simulink model "NovoModeloControlePorPressaoRevFinal_Inter"  (R2017a)
settings: Solver=ode3  StartTime=0.0  StopTime=Tsimulacao  FixedStep=Tamostra  RelTol=1e-3  EnableMultiTasking=on
values from neighbouring files (symbols this model uses):
  Delay = 0.01    [CodigoTeste.m]    (also in CodigoTesteSimulador.m = 1.5; ControlePorPressaoRevFinal.m = input('Escolha o tempo para o delay do ventilador [s] '); PlotsDaSimulacaoFinal.m = 0.05; SimulacaoFinalDaPesquisa.m = ResultadosVentiladorInterrupcaoIntermitente(i,6))
  E = 38.1970    (= 38.197)    [CodigoTeste.m]    (also in CodigoTesteSimulador.m; ControlePorPressaoRevFinal.m = 50; PlotsDaSimulacaoFinal.m = 8.33333333333; SimulacaoFinalDaPesquisa.m = 1/ResultadosVentiladorInterrupcaoIntermitente(i,5))
  Habilitar = 0    [ControlePorPressaoRevFinal.m]    (also in PlotsDaSimulacaoFinal.m = 1; SimulacaoFinalDaPesquisa.m = 1)
  Hz = 1    [ControlePorPressaoRevFinal.m]    (also in PlotsDaSimulacaoFinal.m; SimulacaoFinalDaPesquisa.m = ResultadosVentiladorInterrupcaoIntermitente(i,10))
  Limite_Vazao = 0.5    [CodigoTeste.m]    (also in ControlePorPressaoRevFinal.m = input('Escolha a vazão máxima entregue pelo o ventilador [L/; PlotsDaSimulacaoFinal.m; SimulacaoFinalDaPesquisa.m; Untitled.m = 1)
  Pasp = [-15.2979 -23.3827 -039.5964]    [CodigoTeste.m]    (also in CodigoTesteSimulador.m; ControlePorPressaoRevFinal.m = -200; PlotsDaSimulacaoFinal.m = -200; SimulacaoFinalDaPesquisa.m = -200)
  PressaoDelay = Pvent    (= 5)    [CodigoTeste.m]    (also in CodigoTesteSimulador.m; ControlePorPressaoRevFinal.m = 10; PlotsDaSimulacaoFinal.m = 10; SimulacaoFinalDaPesquisa.m = 10)
  Ptrigger = 0.0    (= 0)    [CodigoTeste.m]    (also in CodigoTesteSimulador.m = 0.5; ControlePorPressaoRevFinal.m = input('Escolha a pressão de trigger do ventilador [cmH2O] '); PlotsDaSimulacaoFinal.m = 0.5; SimulacaoFinalDaPesquisa.m = ResultadosVentiladorInterrupcaoIntermitente(i,7))
  Pvent = 5    [CodigoTeste.m]    (also in CodigoTesteSimulador.m; ControlePorPressaoRevFinal.m = 10; PlotsDaSimulacaoFinal.m = 10; SimulacaoFinalDaPesquisa.m = 10)
  Rrs = 3.3464    [CodigoTeste.m]    (also in CodigoTesteSimulador.m; ControlePorPressaoRevFinal.m = 5; PlotsDaSimulacaoFinal.m = 5; SimulacaoFinalDaPesquisa.m = ResultadosVentiladorInterrupcaoIntermitente(i,4))
  Tamanho_Sonda = 10    [CodigoTeste.m]    (also in CodigoTesteSimulador.m; ControlePorPressaoRevFinal.m = input('Qual o tamanho da sonda utilizada [FR]? 00, 06, 08, 1; PlotsDaSimulacaoFinal.m = 6; SimulacaoFinalDaPesquisa.m = ResultadosVentiladorInterrupcaoIntermitente(i,9))
  TOT = 7.5    [CodigoTeste.m]    (also in CodigoTesteSimulador.m; ControlePorPressaoRevFinal.m = input('Qual o tamanho do Tubo Orotraquial utilizado [mm]? 7.; PlotsDaSimulacaoFinal.m; SimulacaoFinalDaPesquisa.m = ResultadosVentiladorInterrupcaoIntermitente(i,8))
  VolumeInicial = VR+PressaoInicial/E    (= 0.130900332487)    [CodigoTeste.m]    (also in CodigoTesteSimulador.m; ControlePorPressaoRevFinal.m = 1.4; PlotsDaSimulacaoFinal.m = 2.4; SimulacaoFinalDaPesquisa.m = 2.4)
  VR = 0    [CodigoTeste.m]    (also in CodigoTesteSimulador.m; ControlePorPressaoRevFinal.m = 1.2; PlotsDaSimulacaoFinal.m = 1.2; SimulacaoFinalDaPesquisa.m = 1.2)
libraries: simulink x2
settings Model: Creator=Proprietário  LastModifiedBy=Texugão
settings DataIOCC: LimitDataPoints=on  SaveFormat=Array
settings OptimizationCC: LifeSpan=inf
settings DebuggingCC: SolverPrmCheckMsg=warning  SFUnexpectedBacktrackingDiag=warning  SFNoUnconditionalDefaultTransitionDiag=warning  SFExecutionAtInitializationDiag=none
settings HardwareCC: ProdBitPerPointer=32  ProdBitPerSizeT=32  ProdBitPerPtrDiffT=32  ProdLargestAtomicFloat=None  ProdIntDivRoundTo=Undefined  ProdEndianess=Unspecified  ProdWordSize=32  ProdHWDeviceType=32-bit Generic
settings ModelReferenceCC: PropagateSignalLabelsOutOfModel=off
settings GRTTargetCC: TargetLangStandard=C89/C90 (ANSI)  GeneratePreprocessorConditionals=Disable all
settings ConfigComp: CovMetricSettings=dw  CovHtmlReporting=on  CovSaveCumulativeToWorkspaceVar=on  CovSaveSingleToWorkspaceVar=on  CovExternalEMLEnable=off  CovSFcnEnable=off

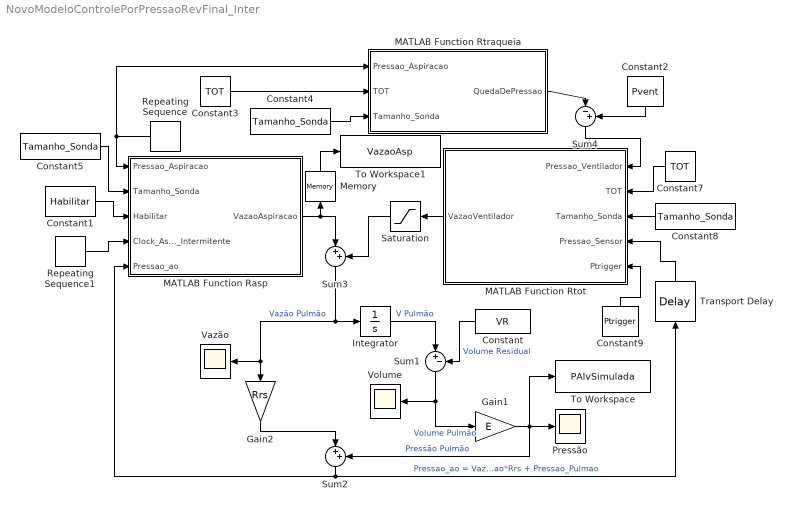
== system NovoModeloControlePorPressaoRevFinal_Inter ==
  Constant : Constant  Value=VR
  Constant1 : Constant  Value=Habilitar
  Constant2 : Constant  Value=Pvent
  Constant3 : Constant  Value=TOT
  Constant4 : Constant  Value=Tamanho_Sonda
  Constant5 : Constant  Value=Tamanho_Sonda
  Constant7 : Constant  Value=TOT
  Constant8 : Constant  Value=Tamanho_Sonda
  Constant9 : Constant  Value=Ptrigger
  Gain1 : Gain  Gain=E
  Gain2 : Gain  Gain=Rrs
  Integrator : Integrator  InitialCondition=VolumeInicial
  MATLAB Function Rasp : MATLAB Function  TreatAsAtomicUnit=on
  MATLAB Function Rtot : MATLAB Function  TreatAsAtomicUnit=on
  MATLAB Function Rtraqueia : MATLAB Function  TreatAsAtomicUnit=on
  Memory : Memory
  Pressão : Scope
  Repeating Sequence : simulink/Sources/Repeating Sequence  rep_seq_t=[0 60 60.001 75 75.001 95]  rep_seq_y=[0 0 Pasp Pasp 0 0]
  Repeating Sequence1 : simulink/Sources/Repeating Sequence  rep_seq_t=[0 1/Hz 1/Hz+0.001 2/Hz]  rep_seq_y=[1 1 0 0]
  Saturation : Saturate  UpperLimit=Limite_Vazao  LowerLimit=-Limite_Vazao
  Sum1 : Sum  Inputs=|+-
  Sum2 : Sum  Inputs=|++
  Sum3 : Sum  Inputs=|++
  Sum4 : Sum  Inputs=|-+
  To Workspace : ToWorkspace  VariableName=PAlvSimulada  SaveFormat=Timeseries  SampleTime=-1
  To Workspace1 : ToWorkspace  VariableName=VazaoAsp  SaveFormat=Timeseries  SampleTime=-1
  Transport Delay : TransportDelay  DelayTime=Delay  InitialOutput=PressaoDelay
  Vazão : Scope
  Volume : Scope
  wires:
  Integrator/1 -> Sum1/1  "V Pulmão"
  Constant/1 -> Sum1/2  "Volume Residual"
  Sum3/1 -> Integrator/1, Vazão/1, Gain2/1  "Vazão Pulmão"
  Sum1/1 -> Gain1/1, Volume/1  "Volume Pulmão"
  Constant5/1 -> MATLAB Function Rasp/2(Tamanho_Sonda)
  Constant8/1 -> MATLAB Function Rtot/3(Tamanho_Sonda)
  Constant7/1 -> MATLAB Function Rtot/2(TOT)
  Transport Delay/1 -> MATLAB Function Rtot/4(Pressao_Sensor)
  Constant9/1 -> MATLAB Function Rtot/5(Ptrigger)
  MATLAB Function Rasp/1(VazaoAspiracao) -> Sum3/1, Memory/1
  Gain1/1 -> To Workspace/1, Pressão/1, Sum2/2  "Pressão Pulmão"
  Gain2/1 -> Sum2/1
  Sum2/1 -> MATLAB Function Rasp/5(Pressao_ao), Transport Delay/1  "Pressao_ao = Vazao_Pulmao*Rrs + Pressao_Pulmao"
  MATLAB Function Rtot/1(VazaoVentilador) -> Saturation/1
  Saturation/1 -> Sum3/2
  Repeating Sequence/1 -> MATLAB Function Rtraqueia/1(Pressao_Aspiracao), MATLAB Function Rasp/1(Pressao_Aspiracao)
  Constant1/1 -> MATLAB Function Rasp/3(Habilitar)
  Repeating Sequence1/1 -> MATLAB Function Rasp/4(Clock_Aspiracao_Intermitente)
  Constant4/1 -> MATLAB Function Rtraqueia/3(Tamanho_Sonda)
  Constant3/1 -> MATLAB Function Rtraqueia/2(TOT)
  Sum4/1 -> MATLAB Function Rtot/1(Pressao_Ventilador)
  Constant2/1 -> Sum4/2
  MATLAB Function Rtraqueia/1(QuedaDePressao) -> Sum4/1
  Memory/1 -> To Workspace1/1

== matlab function NovoModeloControlePorPressaoRevFinal_Inter/MATLAB Function Rtraqueia ==
  data: Pressao_Aspiracao input; TOT input; Tamanho_Sonda input; QuedaDePressao output
function QuedaDePressao = Interferencia(Pressao_Aspiracao, TOT, Tamanho_Sonda)


%Estimação da Vazão de acordo com a combinação de TOT [7.5 ou 8.5] e Tamanho da Sonda utilizada [06, 08, 10, ou 12]
DeltaP = 1;
if TOT == 7.5
    if Tamanho_Sonda == 06
        DeltaP = -0.00235*Pressao_Aspiracao+0.2535;
    elseif Tamanho_Sonda == 08
        DeltaP = -0.01294*Pressao_Aspiracao+0.1899;
    elseif Tamanho_Sonda == 10
        DeltaP = -0.03382*Pressao_Aspiracao+0.9449;
    end
elseif TOT == 8.5
    if Tamanho_Sonda == 06
        DeltaP = -0.009146*Pressao_Aspiracao+0.3947;
    elseif Tamanho_Sonda == 08
        DeltaP = -0.03089*Pressao_Aspiracao+0.8912;
    elseif Tamanho_Sonda == 10
        DeltaP = -0.05433*Pressao_Aspiracao+0.9346;
    elseif Tamanho_Sonda == 12
        DeltaP = -0.06652*Pressao_Aspiracao+1.668;
    end
end

QuedaDePressao = DeltaP;

end

== matlab function NovoModeloControlePorPressaoRevFinal_Inter/MATLAB Function Rasp ==
  data: Pressao_Aspiracao input; Tamanho_Sonda input; Habilitar input; Clock_Aspiracao_Intermitente input; Pressao_ao input; VazaoAspiracao output
function VazaoAspiracao = VazaoAspiracao(Pressao_Aspiracao, Tamanho_Sonda,Habilitar,Clock_Aspiracao_Intermitente, Pressao_ao)

%Bug do Simulink está tratando os sinais como complexos. 
%Então se trabalha com o modulo
Delta_P = abs(Pressao_Aspiracao - Pressao_ao);

%Correção do sinal pelo o Bug
Sinal = 1;
if Pressao_Aspiracao < Pressao_ao
    %Pressão Aspiração mais negativa que o paciente
    Sinal = -1;
else
    %Pressão do paciente mais negativa que a pressão Aspiração
    Sinal = 1;
end

%Estimação da Vazão de acordo com o Tamanho da Sonda utilizada [00, 06, 08, 10, ou 12]
Vazao = 1;
Rasp = 1;
if Tamanho_Sonda == 0
    Vazao = 0;
elseif Tamanho_Sonda == 06
    Vazao = 0.001339*Delta_P^0.7939;   
elseif Tamanho_Sonda == 08
    Vazao = 0.01081*Delta_P^0.6338;
elseif Tamanho_Sonda == 10
    Vazao = 0.01501*Delta_P^0.6046;
elseif Tamanho_Sonda == 12
    Vazao = 0.03048*Delta_P^0.5689;
elseif Tamanho_Sonda == 14
    Vazao = 0.05087*Delta_P^0.5644;
end

%Aspiração Intermitente
if Habilitar == 1 %Permitiu
    if Clock_Aspiracao_Intermitente == 0 %Clock para parar de aspirar
        Vazao = 0; %Parou de aspirar
    end        
end

VazaoAspiracao = Sinal*Vazao;

end

== matlab function NovoModeloControlePorPressaoRevFinal_Inter/MATLAB Function Rtot ==
  data: Pressao_Ventilador input; TOT input; Tamanho_Sonda input; Pressao_Sensor input; VazaoVentilador output; Ptrigger input
function VazaoVentilador = VazaoVentilador(Pressao_Ventilador, TOT, Tamanho_Sonda, Pressao_Sensor, Ptrigger)

%Bug do Simulink está tratando os sinais como complexos. 
%Então se trabalha com o modulo
Delta_P = abs(Pressao_Ventilador - Pressao_Sensor);

%Correção do sinal pelo o Bug
Sinal = 1;
if Pressao_Ventilador < Pressao_Sensor
    %Pressao do ventilador menor que a pressão do paciente
    Sinal = -1;
else
    Sinal = 1;
end

%Sensibilidade do Ventilador
persistent Status_Ventilador; %A variável Status_Ventilador mantem o valor entre execuções
if isempty(Status_Ventilador)
    %Se está vazio, começa desligado
    Status_Ventilador=false;
end
if Delta_P == 0     
    %Desliga o Ventilador
    Status_Ventilador = false;
elseif Delta_P > Ptrigger
    %Ativa o ventilador
    Status_Ventilador = true;
end

if Status_Ventilador
    %Mantem o Delta_P
else
    %Se o ventilador desligado, não tem vazão
    Delta_P =0;
end 

%Estimação da Vazão de acordo com a combinação de TOT [7.5 ou 8.5] e Tamanho da Sonda utilizada [00, 06, 08, 10, ou 12]
Vazao = 1;
Rtot = 1;
if TOT == 7.5
    if Tamanho_Sonda == 0
        Vazao = 0.3833*Delta_P^0.5872;
    elseif Tamanho_Sonda == 06
        Vazao = 0.3223*Delta_P^0.5745;
    elseif Tamanho_Sonda == 08
        Vazao = 0.2745*Delta_P^0.5687;
    elseif Tamanho_Sonda == 10
        Vazao = 0.2682*Delta_P^0.5726;
    end
elseif TOT == 8.5
    if Tamanho_Sonda == 0
        Vazao = 0.548*Delta_P^0.5688;
    elseif Tamanho_Sonda == 06
        Vazao = 0.4413*Delta_P^0.5807;
    elseif Tamanho_Sonda == 08
        Vazao = 0.3795*Delta_P^0.5819;
    elseif Tamanho_Sonda == 10
        Vazao = 0.3808*Delta_P^0.5843;
    elseif Tamanho_Sonda == 12
        Vazao = 0.321*Delta_P^0.5871;
    end
end

VazaoVentilador = Sinal*Vazao;

end
